simulink model "All_injectors_with_LQG"  (R2022a)
settings: Solver=FixedStepAuto  StartTime=0.0  StopTime=.004  FixedStep=SampleTime  RelTol=1e-3
values from neighbouring files (symbols this model uses):
  A = (state_derivative_coeff) \ state_coeff    [All_injectors_LQG_bop_ss_model_code.m]    (also in All_injectors_LQG_continuous_time_code.m; All_injectors_LQG_plasma_7_15_24_code.m; All_injectors_LQG_plasma_ss_model_code.m; All_injectors_vaccum.m = sysc.A)
  Ad = sys_d_plasma.A    [All_injectors_LQG_bop_plasma_ss_model_code.m]    (also in All_injectors_LQG_bop_ss_model_code.m; All_injectors_LQG_continuous_time_code.m; All_injectors_LQG_plasma_7_15_24_code.m; All_injectors_LQG_plasma_ss_model_code.m)
  Amplitude = 600    [All_injectors_LQG_bop_plasma_ss_model_code.m]    (also in All_injectors_LQG_bop_ss_model_code.m; All_injectors_LQG_continuous_time_code.m; All_injectors_LQG_plasma_7_15_24_code.m; All_injectors_LQG_plasma_ss_model_code.m)
  Amplitude1 = 600    [All_injectors_vaccum.m]    (also in All_injectors_with_LQG_code.m; MPC_attempt.m; Plasma_ss_model.m; Use_for_freq_scan.m)
  Bd = sys_d_plasma.B    [All_injectors_LQG_bop_plasma_ss_model_code.m]    (also in All_injectors_LQG_bop_ss_model_code.m; All_injectors_LQG_continuous_time_code.m; All_injectors_LQG_plasma_7_15_24_code.m; All_injectors_LQG_plasma_ss_model_code.m)
  Cap = 96e-6    (= 9.6e-05)    [All_injectors_LQG_bop_ss_model_code.m]    (also in All_injectors_LQG_continuous_time_code.m; All_injectors_LQG_plasma_7_15_24_code.m; All_injectors_LQG_plasma_ss_model_code.m; All_injectors_vaccum.m)
  Cd = sys_d_plasma.C    [All_injectors_LQG_bop_plasma_ss_model_code.m]    (also in All_injectors_LQG_bop_ss_model_code.m; All_injectors_LQG_continuous_time_code.m; All_injectors_LQG_plasma_7_15_24_code.m; All_injectors_LQG_plasma_ss_model_code.m)
  Dd = sys_d_plasma.D    [All_injectors_LQG_bop_plasma_ss_model_code.m]    (also in All_injectors_LQG_bop_ss_model_code.m; All_injectors_LQG_continuous_time_code.m; All_injectors_LQG_plasma_7_15_24_code.m; All_injectors_LQG_plasma_ss_model_code.m)
  desired_L2_amplitude = 10000    [All_injectors_with_LQG_code.m]
  Frequency = 19000    [All_injectors_LQG_bop_plasma_ss_model_code.m]    (also in All_injectors_LQG_bop_ss_model_code.m; All_injectors_LQG_continuous_time_code.m; All_injectors_LQG_plasma_7_15_24_code.m; All_injectors_LQG_plasma_ss_model_code.m)
  L1 = (9.78e-7)    (= 9.78e-07)    [All_injectors_LQG_bop_plasma_ss_model_code.m]    (also in All_injectors_LQG_bop_ss_model_code.m = 8.0141e-07; All_injectors_LQG_continuous_time_code.m = 8.0141e-07; All_injectors_LQG_plasma_7_15_24_code.m = 8.0141e-07; All_injectors_LQG_plasma_ss_model_code.m = 8.0141e-07)
  L2 = 2.0462e-6    (= 2.0462e-06)    [All_injectors_LQG_bop_ss_model_code.m]    (also in All_injectors_LQG_continuous_time_code.m; All_injectors_LQG_plasma_7_15_24_code.m; All_injectors_LQG_plasma_ss_model_code.m; All_injectors_vaccum.m)
  Lp = L2    (= 2.0462e-06)    [All_injectors_LQG_bop_ss_model_code.m]    (also in All_injectors_LQG_continuous_time_code.m; All_injectors_LQG_plasma_7_15_24_code.m; All_injectors_LQG_plasma_ss_model_code.m; Plasma_ss_model.m = 1.0231e-06)
  M = .161*L2    (= 3.294382e-07)    [All_injectors_LQG_bop_ss_model_code.m]    (also in All_injectors_LQG_continuous_time_code.m; All_injectors_LQG_plasma_7_15_24_code.m; All_injectors_LQG_plasma_ss_model_code.m; All_injectors_vaccum.m)
  Mw = .1346*L2    (= 2.7541852e-07)    [All_injectors_LQG_bop_ss_model_code.m]    (also in All_injectors_LQG_continuous_time_code.m; All_injectors_LQG_plasma_7_15_24_code.m; All_injectors_LQG_plasma_ss_model_code.m; All_injectors_vaccum.m)
  NoisePower = 0    [All_injectors_LQG_bop_plasma_ss_model_code.m]    (also in All_injectors_LQG_bop_ss_model_code.m = 0.0001; All_injectors_LQG_continuous_time_code.m = 0.0001; All_injectors_LQG_plasma_7_15_24_code.m; All_injectors_LQG_plasma_ss_model_code.m = 0.0001)
  R = 1    [All_injectors_LQG_bop_plasma_ss_model_code.m]    (also in All_injectors_LQG_bop_ss_model_code.m = diag(1*ones(1,num_inputs)); All_injectors_LQG_continuous_time_code.m = diag(1*ones(1,num_inputs)); All_injectors_LQG_plasma_7_15_24_code.m = diag(1*ones(1,num_inputs)); All_injectors_LQG_plasma_ss_model_code.m = diag(1*ones(1,num_inputs)))
  R1 = .0025    (= 0.0025)    [All_injectors_LQG_bop_ss_model_code.m]    (also in All_injectors_LQG_continuous_time_code.m; All_injectors_LQG_plasma_7_15_24_code.m; All_injectors_LQG_plasma_ss_model_code.m; All_injectors_vaccum.m)
  R2 = .005    (= 0.005)    [All_injectors_LQG_bop_ss_model_code.m]    (also in All_injectors_LQG_continuous_time_code.m; All_injectors_LQG_plasma_7_15_24_code.m; All_injectors_LQG_plasma_ss_model_code.m; All_injectors_vaccum.m)
  R3 = .005    (= 0.005)    [All_injectors_LQG_bop_ss_model_code.m]    (also in All_injectors_LQG_continuous_time_code.m; All_injectors_LQG_plasma_7_15_24_code.m; All_injectors_LQG_plasma_ss_model_code.m; All_injectors_vaccum.m)
  RunTime = .004    (= 0.004)    [All_injectors_LQG_bop_plasma_ss_model_code.m]    (also in All_injectors_LQG_bop_ss_model_code.m; All_injectors_LQG_continuous_time_code.m; All_injectors_LQG_plasma_7_15_24_code.m; All_injectors_LQG_plasma_ss_model_code.m)
  SampleTime = 1e-7    (= 1e-07)    [All_injectors_LQG_bop_plasma_ss_model_code.m]    (also in All_injectors_LQG_bop_ss_model_code.m; All_injectors_LQG_continuous_time_code.m; All_injectors_LQG_plasma_7_15_24_code.m; All_injectors_LQG_plasma_ss_model_code.m)
  voltage = Amplitude*sin(2*pi*Frequency*time)    [All_injectors_LQG_bop_plasma_ss_model_code.m]    (also in All_injectors_LQG_bop_ss_model_code.m; All_injectors_LQG_continuous_time_code.m; All_injectors_LQG_plasma_7_15_24_code.m; All_injectors_LQG_plasma_ss_model_code.m)
undefined symbols (not defined in the file or in its folder): Discrete, K, L1_V, Time
libraries: spsSeriesRLCBranchLib x50, simulink x23, spsCurrentMeasurementLib x20, spsDCVoltageSourceLib x12, spsVoltageMeasurementLib x12, spsFullBridgeMMCExternalDCLinksLib x9, spsPWMGeneratorMultilevelLib x9, ctrlSharedLib x6, spsMosfetLib x4, spsParallelRLCBranchLib x2, spsMutualInductanceLib x1, spspowerguiLib x1
(part 2 of 2)

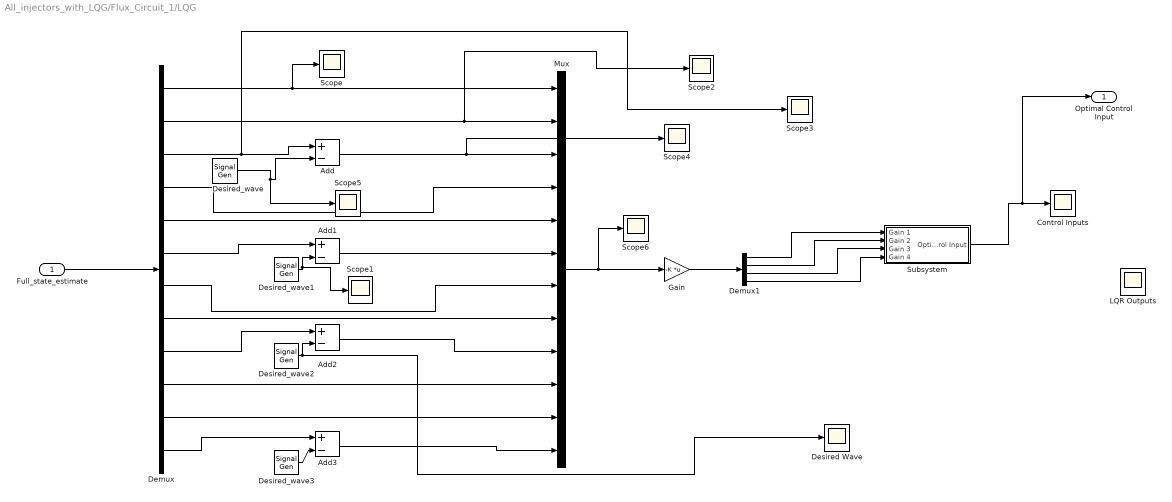
== system All_injectors_with_LQG/Flux_Circuit_1/LQG ==
  Full_state_estimate : Inport
  Add{,1..3} (4 alike) : Sum  Inputs=+-
  Control Inputs : Scope
  Demux : Demux  Outputs=size(A,1)
  Demux1 : Demux  Outputs=4.
  Desired Wave : Scope
  Desired_wave{,1..3} (4 alike) : SignalGenerator  Amplitude=desired_L2_amplitude  Frequency=Frequency
  Gain : Gain  Gain=-K  Multiplication=Matrix(K*u) (u vector)
  LQR Outputs : Scope
  Mux : Mux  Inputs=size(A,1)
  Scope{,1..6} (7 alike) : Scope
  Subsystem : Subsystem
  Optimal Control Input : Outport
  wires:
  Full_state_estimate/1 -> Demux/1
  Demux/1 -> Scope/1, Mux/1
  Demux/2 -> Scope2/1, Mux/2
  Demux/3 -> Scope3/1, Add/1
  Desired_wave/1 -> Scope5/1, Add/2
  Add/1 -> Scope4/1, Mux/3
  Demux/4 -> Mux/4
  Demux/5 -> Mux/5
  Demux/6 -> Add1/1
  Add1/1 -> Mux/6
  Desired_wave1/1 -> Scope1/1, Add1/2
  Demux/7 -> Mux/7
  Demux/8 -> Mux/8
  Desired_wave2/1 -> Add2/2, Desired Wave/1
  Demux/9 -> Add2/1
  Add2/1 -> Mux/9
  Demux/10 -> Mux/10
  Demux/11 -> Mux/11
  Desired_wave3/1 -> Add3/2
  Demux/12 -> Add3/1
  Add3/1 -> Mux/12
  Gain/1 -> Demux1/1
  Demux1/1 -> Subsystem/1(Gain 1)
  Demux1/2 -> Subsystem/2(Gain 2)
  Demux1/3 -> Subsystem/3(Gain 3)
  Demux1/4 -> Subsystem/4("Gain 4 ")
  Subsystem/1(Optimal Control Input) -> Optimal Control Input/1, Control Inputs/1
  Mux/1 -> Scope6/1, Gain/1

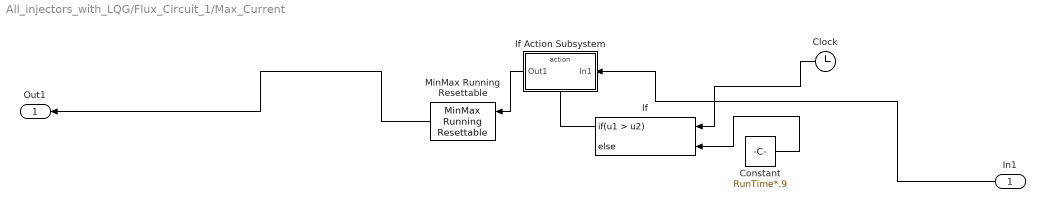
== system All_injectors_with_LQG/Flux_Circuit_1/Max_Current ==
  In1 : Inport
  Clock : Clock
  Constant : Constant  Value=RunTime*.9
  If : If  NumInputs=2  IfExpression=u1 > u2
  If Action Subsystem : Subsystem  TreatAsAtomicUnit=on
  MinMax Running Resettable : simulink/Math Operations/MinMax Running Resettable  Function=max  vinit=0.0
  Out1 : Outport
  wires:
  In1/1 -> If Action Subsystem/1(In1)
  If Action Subsystem/1(Out1) -> MinMax Running Resettable/1
  MinMax Running Resettable/1 -> Out1/1
  Constant/1 -> If/2
  Clock/1 -> If/1
  If/1 -> If Action Subsystem/Action

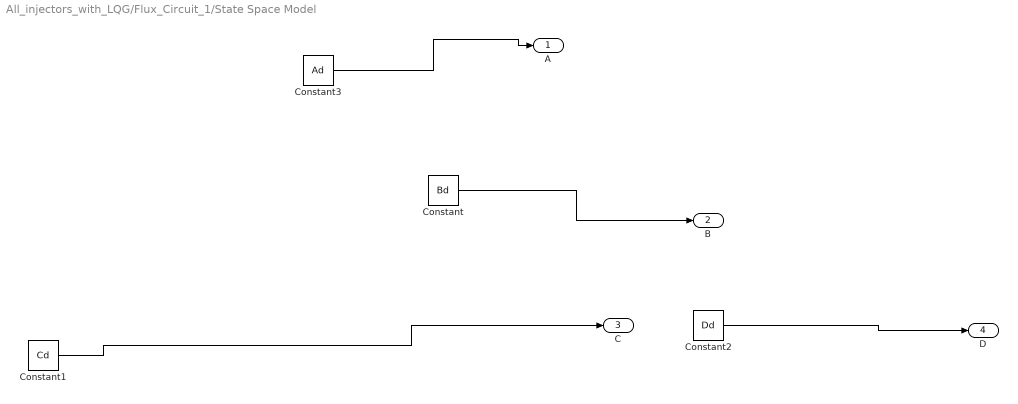
== system All_injectors_with_LQG/Flux_Circuit_1/State Space Model ==
  Constant : Constant  Value=Bd
  Constant1 : Constant  Value=Cd
  Constant2 : Constant  Value=Dd
  Constant3 : Constant  Value=Ad
  A : Outport
  B : Outport  Port=2
  C : Outport  Port=3
  D : Outport  Port=4
  wires:
  Constant3/1 -> A/1
  Constant2/1 -> D/1
  Constant/1 -> B/1
  Constant1/1 -> C/1

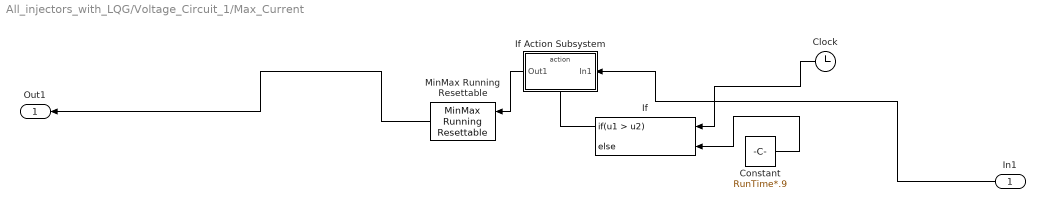
== system All_injectors_with_LQG/Voltage_Circuit_1/Max_Current ==
  In1 : Inport
  Clock : Clock
  Constant : Constant  Value=RunTime*.9
  If : If  NumInputs=2  IfExpression=u1 > u2
  If Action Subsystem : Subsystem  TreatAsAtomicUnit=on
  MinMax Running Resettable : simulink/Math Operations/MinMax Running Resettable  Function=max  vinit=0.0
  Out1 : Outport
  wires:
  In1/1 -> If Action Subsystem/1(In1)
  If Action Subsystem/1(Out1) -> MinMax Running Resettable/1
  MinMax Running Resettable/1 -> Out1/1
  Constant/1 -> If/2
  Clock/1 -> If/1
  If/1 -> If Action Subsystem/Action

== system All_injectors_with_LQG/Voltage_Circuit_2/Max_Current ==
  In1 : Inport
  Clock : Clock
  Constant : Constant  Value=RunTime*.9
  If : If  NumInputs=2  IfExpression=u1 > u2
  If Action Subsystem : Subsystem  TreatAsAtomicUnit=on
  MinMax Running Resettable : simulink/Math Operations/MinMax Running Resettable  Function=max  vinit=0.0
  Out1 : Outport
  wires:
  In1/1 -> If Action Subsystem/1(In1)
  If Action Subsystem/1(Out1) -> MinMax Running Resettable/1
  MinMax Running Resettable/1 -> Out1/1
  Constant/1 -> If/2
  Clock/1 -> If/1
  If/1 -> If Action Subsystem/Action

== system All_injectors_with_LQG/Voltage_Circuit_3/Max_Current ==
  In1 : Inport
  Clock : Clock
  Constant : Constant  Value=RunTime*.9
  If : If  NumInputs=2  IfExpression=u1 > u2
  If Action Subsystem : Subsystem  TreatAsAtomicUnit=on
  MinMax Running Resettable : simulink/Math Operations/MinMax Running Resettable  Function=max  vinit=0.0
  Out1 : Outport
  wires:
  In1/1 -> If Action Subsystem/1(In1)
  If Action Subsystem/1(Out1) -> MinMax Running Resettable/1
  MinMax Running Resettable/1 -> Out1/1
  Constant/1 -> If/2
  Clock/1 -> If/1
  If/1 -> If Action Subsystem/Action

== system All_injectors_with_LQG/Voltage_Circuit_4/Max_Current ==
  In1 : Inport
  Clock : Clock
  Constant : Constant  Value=RunTime*.9
  If : If  NumInputs=2  IfExpression=u1 > u2
  If Action Subsystem : Subsystem  TreatAsAtomicUnit=on
  MinMax Running Resettable : simulink/Math Operations/MinMax Running Resettable  Function=max  vinit=0.0
  Out1 : Outport
  wires:
  In1/1 -> If Action Subsystem/1(In1)
  If Action Subsystem/1(Out1) -> MinMax Running Resettable/1
  MinMax Running Resettable/1 -> Out1/1
  Constant/1 -> If/2
  Clock/1 -> If/1
  If/1 -> If Action Subsystem/Action

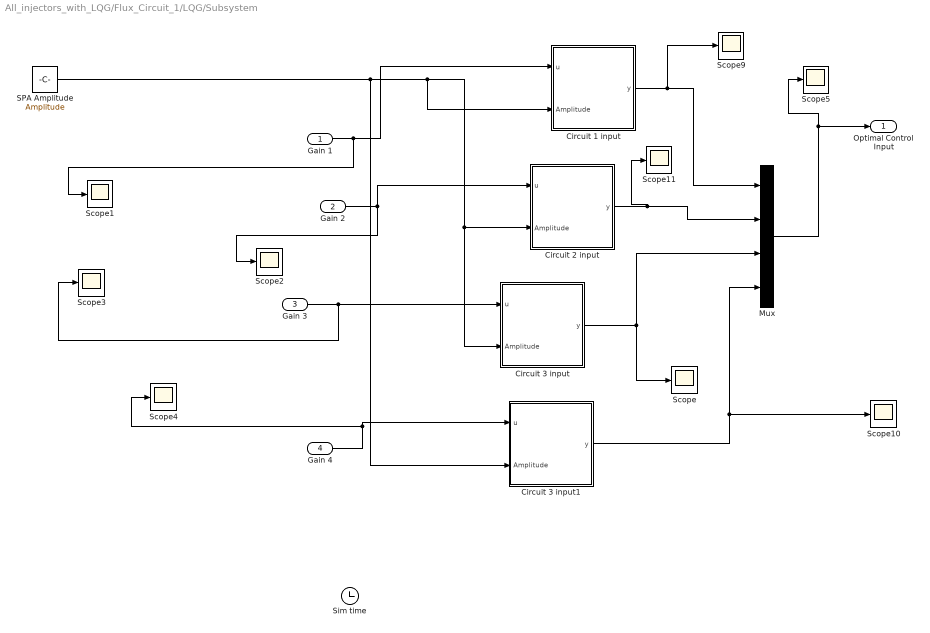
== system All_injectors_with_LQG/Flux_Circuit_1/LQG/Subsystem ==
  Gain 1 : Inport
  Gain 2 : Inport  Port=2
  Gain 3 : Inport  Port=3
  "Gain 4 " : Inport  Port=4
  Circuit 1 input : MATLAB Function  TreatAsAtomicUnit=on
  Circuit 2 input : MATLAB Function  TreatAsAtomicUnit=on
  Circuit 3 input : MATLAB Function  TreatAsAtomicUnit=on
  Circuit 3 input1 : MATLAB Function  TreatAsAtomicUnit=on
  Mux : Mux
  SPA Amplitude : Constant  Value=Amplitude
  Scope{,1..5,9..11} (9 alike) : Scope
  Sim time : Clock
      settings: Decimation=100000
  Optimal Control Input : Outport
  wires:
  Gain 2/1 -> Circuit 2 input/1(u), Scope2/1
  Circuit 3 input/1(y) -> Scope/1, Mux/3
  "Gain 4 "/1 -> Circuit 3 input1/1(u), Scope4/1
  Mux/1 -> Scope5/1, Optimal Control Input/1
  Gain 3/1 -> Scope3/1, Circuit 3 input/1(u)
  SPA Amplitude/1 -> Circuit 3 input1/2(Amplitude), Circuit 1 input/2(Amplitude), Circuit 3 input/2(Amplitude), Circuit 2 input/2(Amplitude)
  Gain 1/1 -> Scope1/1, Circuit 1 input/1(u)
  Circuit 1 input/1(y) -> Scope9/1, Mux/1
  Circuit 2 input/1(y) -> Scope11/1, Mux/2
  Circuit 3 input1/1(y) -> Scope10/1, Mux/4

== system All_injectors_with_LQG/Flux_Circuit_1/Max_Current/If Action Subsystem ==
  In1 : Inport
  Action Port : ActionPort  ActionPortLabel=if(u1 > u2)
  Out1 : Outport
  wires:
  In1/1 -> Out1/1

== system All_injectors_with_LQG/Voltage_Circuit_1/Max_Current/If Action Subsystem ==
  In1 : Inport
  Action Port : ActionPort  ActionPortLabel=if(u1 > u2)
  Out1 : Outport
  wires:
  In1/1 -> Out1/1

== system All_injectors_with_LQG/Voltage_Circuit_2/Max_Current/If Action Subsystem ==
  In1 : Inport
  Action Port : ActionPort  ActionPortLabel=if(u1 > u2)
  Out1 : Outport
  wires:
  In1/1 -> Out1/1

== system All_injectors_with_LQG/Voltage_Circuit_3/Max_Current/If Action Subsystem ==
  In1 : Inport
  Action Port : ActionPort  ActionPortLabel=if(u1 > u2)
  Out1 : Outport
  wires:
  In1/1 -> Out1/1

== system All_injectors_with_LQG/Voltage_Circuit_4/Max_Current/If Action Subsystem ==
  In1 : Inport
  Action Port : ActionPort  ActionPortLabel=if(u1 > u2)
  Out1 : Outport
  wires:
  In1/1 -> Out1/1

== matlab function All_injectors_with_LQG/Flux_Circuit_1/LQG/Subsystem/Circuit 2 input ==
  data: u input double size=[1,1]; y output double size=[1,1]; Amplitude input
function y = convert_to_square(u,Amplitude)

d1 = abs(Amplitude-u);
d2 = abs(u);
d3 = abs(-Amplitude-u);
if min([d1,d2,d3]) == d1
    y = Amplitude;
elseif min([d1,d2,d3]) == d2
    y = 0;
else 
    y = -Amplitude;
end
%y = u;

== matlab function All_injectors_with_LQG/Flux_Circuit_1/LQG/Subsystem/Circuit 3 input1 ==
  data: u input double size=[1,1]; y output double size=[1,1]; Amplitude input
function y = convert_to_square(u,Amplitude)

d1 = abs(Amplitude-u);
d2 = abs(u);
d3 = abs(-Amplitude-u);
if min([d1,d2,d3]) == d1
    y = Amplitude;
elseif min([d1,d2,d3]) == d2
    y = 0;
else 
    y = -Amplitude;
end
%y = u;

== matlab function All_injectors_with_LQG/Flux_Circuit_1/LQG/Subsystem/Circuit 3 input ==
  data: u input double size=[1,1]; y output double size=[1,1]; Amplitude input
function y = convert_to_square(u,Amplitude)

d1 = abs(Amplitude-u);
d2 = abs(u);
d3 = abs(-Amplitude-u);
if min([d1,d2,d3]) == d1
    y = Amplitude;
elseif min([d1,d2,d3]) == d2
    y = 0;
else 
    y = -Amplitude;
end
%y = u;

== matlab function All_injectors_with_LQG/Flux_Circuit_1/LQG/Subsystem/Circuit 1 input ==
  data: u input double size=[1,1]; y output double size=[1,1]; Amplitude input
function y = convert_to_square(u,Amplitude)

d1 = abs(Amplitude-u);
d2 = abs(u);
d3 = abs(-Amplitude-u);
if min([d1,d2,d3]) == d1
    y = Amplitude;
elseif min([d1,d2,d3]) == d2
    y = 0;
else 
    y = -Amplitude;
end
%y = u;
